simulink library "IOlib"  (R2014a)
settings: Solver=ode45  SolverMode=SingleTasking  StartTime=0.0  StopTime=10.0  RelTol=1e-3
values from neighbouring files (symbols this model uses):
  tm = (tm_l + tm_r)./2    [AACplottingcode.m]    (also in AACplottingcode_Mzcurves.m = 0.0212; IMECE06plottingcode.m; If_alpha_tp_observer_shoreline.m)
  Ts = 0.002    [DSC_Control_Analysis.m]    (also in DSC_Control_Analysis_Exp.m; DSC_Speed_Control_Analysis.m; EC_params_nissan.m; Ext_MPCPara.m = SSD.Ts)
undefined symbols (not defined in the file or in its folder): Amps_per_volt, bs, Eff, eff, fs, gr, Js, Kf, Ki, kM, Kp, L, ljt, lma, lmt, lsa, R, rjt, rma, rmt, rsa
undefined symbols (not defined in the file): DataDescription
libraries: simulink x3, xpcdiamondlib x2, HardwareIO x2, NullHardware x1, PrerecordData x1, VehicleSimulation x1
(part 1 of 2)
settings Model: ExtModeAutoUpdateStatusClock=off  Creator=cgadda  LastModifiedBy=cbeal

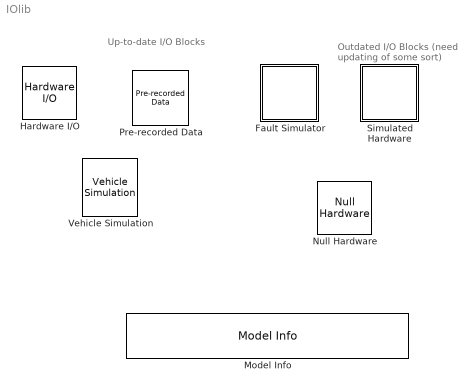
== system IOlib ==
  note: Up-to-date I/O Blocks
  note: Outdated I/O Blocks
      | (need updating of some sort)
  Fault Simulator : Subsystem
      mask init:
      | set_param('nissan_steer','StopTime','36000');
      | set_param('nissan_steer','StartTime','0');
      settings: OpenFcn=open_system([gcb '/Fault Simulator']);
      mask Display: disp('xPC');
  Hardware I/O : HardwareIO/Hardware I//O
  Model Info : simulink/Model-Wide Utilities/Model Info  InitialBlockCM=cvs  BlockCM=cvs  Frame=off  DisplayStringWithTags=|  HorizontalTextAlignment=Left  LeftAlignmentValue=0.02  SourceBlockDiagram=IOlib  TagMaxNumber=20
      | Last saved on: %<LastModificationDate>
      | Save number: %<ModelVersion>
      | Subversion: $Revision: 473 $
  Null Hardware : NullHardware/Null Hardware  SystemSampleTime=-1
  Pre-recorded Data : PrerecordData/Pre-recorded Data  filename=beal_2005-12-06_ab.mat  timeflag=off  starttime=0  stoptime=0
  Simulated Hardware : Subsystem  mask{stepsize=100, v=10, UseRealData=on, filename=/users/cgadda/nissan test data/Moffett1/gerdes_2004-12-11_a.mat}
      mask prompts: stepsize "Handwheel step steer magnitude (deg):"; v "Vehicle speed:"; UseRealData "Use pre-recorded driver input:"; filename "Pre-recorded data filename:"
      mask help:
      | This block provides a simulated hardware model.
      |
      | The driver command (speed and handwheel angle) is a step steer at constant speed.  The speed and magnitude of the manuever can be specified below.  Alternatively, the driver command can be taken from a pre-recorded data file.
      |
      | Note: when using this block, you MUST use a variable step size solver such as ode23.
      mask init:
      | p1_params
      | 
      | if(strcmp(filename,'-')|~UseRealData)
      | 	y=ones(1,18);
      | 	t=0;
      | 	DataDescription(1).name='Handwheel';
      | 	DataDescription(1).size=1;
      | 	DataDescription(2).name='GPS';
      | 	DataDescription(2).size=17;
      | else
      | 	load(filename);
      | end
      | 	
      | if(~(exist('DataDescription')&exist('y')&exist('t')))
      | 	error('Invalid data file.');
      | end
      mask Callback UseRealData:
      | if(strcmp(get_param(gcbh,'UseRealData'),'on')),
      | 	set_param(gcbh,'MaskEnables',{'off' 'off' 'on' 'on'});
      | else
      | 	set_param(gcbh,'MaskEnables',{'on' 'on' 'on' 'off'});
      | end
      mask Display: disp('Sim');
  Vehicle Simulation : VehicleSimulation/Vehicle Simulation  InitPosE=0  InitPosN=0  InitYawAngle=0  CruiseEnableTime=1  AutoSteerEnable=on  FaultEnable=off  HWHALEnable=off  TwoWheelEnable=on  DiffDriveEnable=off

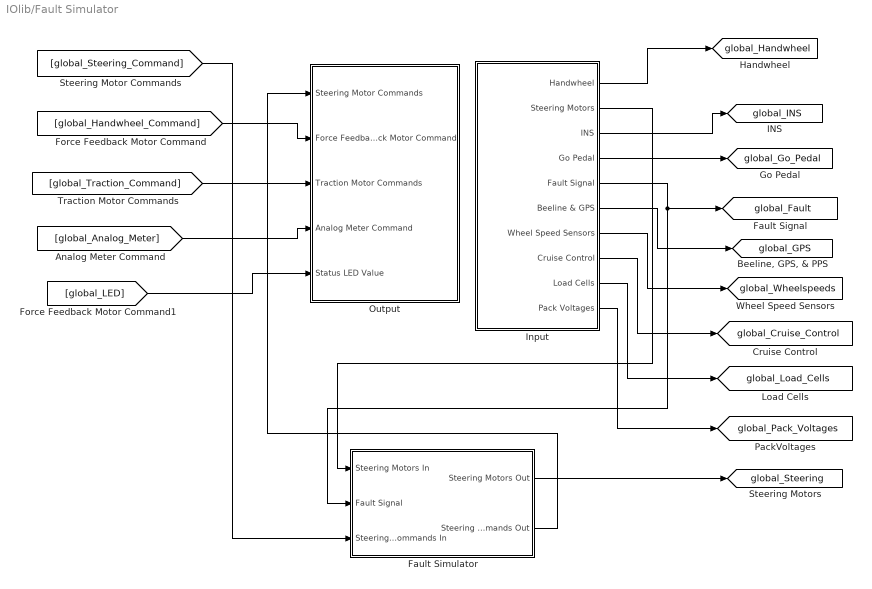
== system IOlib/Fault Simulator ==
  Fault Simulator : Subsystem  mask{fault=Current sensor, magnitude=0}
      mask prompts: fault "Type of fault"
      mask init:
      | switch(fault)
      | 	case 1
      | 		current=magnitude;
      | 		steer=0;
      | 	case 2
      | 		current=0;
      | 		steer=magnitude;
      | end
      mask TypeOptions fault: Current sensor | Steer angle sensor
  Input : Subsystem
  Output : Subsystem
  tag scope: global_Cruise_Control=global, global_Fault=global, global_GPS=global, global_Go_Pedal=global, global_Handwheel=global, global_INS=global, global_Load_Cells=global, global_Pack_Voltages=global, global_Steering=global, global_Wheelspeeds=global
  wires:
  Input/10(Pack Voltages) -> [global_Pack_Voltages]
  Input/9(Load Cells) -> [global_Load_Cells]
  [global_Traction_Command] -> Output/3(Traction Motor Commands)
  [global_Analog_Meter] -> Output/4(Analog Meter Command)
  [global_Steering_Command] -> Fault Simulator/3(Steering Motor Commands In)
  [global_Handwheel_Command] -> Output/2(Force Feedback Motor Command)
  [global_LED] -> Output/5(Status LED Value)
  Input/1(Handwheel) -> [global_Handwheel]
  Input/2(Steering Motors) -> Fault Simulator/1(Steering Motors In)
  Input/3(INS) -> [global_INS]
  Input/4(Go Pedal) -> [global_Go_Pedal]
  Input/5(Fault Signal) -> [global_Fault], Fault Simulator/2(Fault Signal)
  Input/6(Beeline & GPS) -> [global_GPS]
  Input/7(Wheel Speed Sensors) -> [global_Wheelspeeds]
  Input/8(Cruise Control) -> [global_Cruise_Control]
  Fault Simulator/1(Steering Motors Out) -> [global_Steering]
  Fault Simulator/2(Steering Motor Commands Out) -> Output/1(Steering Motor Commands)

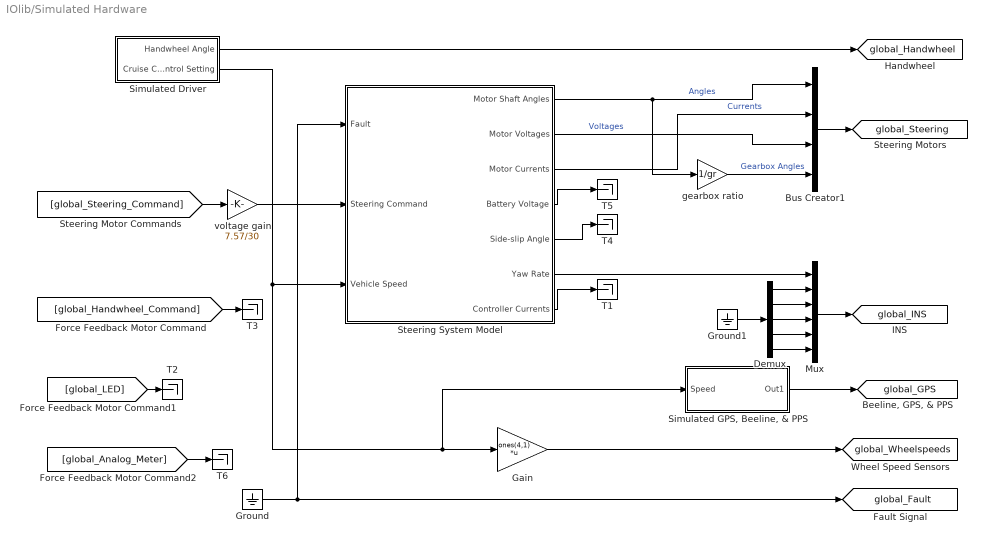
== system IOlib/Simulated Hardware ==
  Bus Creator1 : BusCreator
  Demux : Demux  Outputs=5
  Gain : Gain  Gain=ones(4,1)  Multiplication=Matrix(K*u)  SaturateOnIntegerOverflow=on  OutDataTypeStr=Inherit: Same as input  ParamDataTypeStr=Inherit: Same as input
  Ground : Ground
  Ground1 : Ground
  Mux : Mux  Inputs=6
  Simulated Driver : Subsystem
  "Simulated GPS, Beeline, & PPS" : Subsystem
  Steering System Model : Subsystem
  T{1..6} (6 alike) : Terminator
  gearbox ratio : Gain  Gain=1/gr  SaturateOnIntegerOverflow=on  OutDataTypeStr=Inherit: Same as input  ParamDataTypeStr=Inherit: Same as input
  voltage gain : Gain  Gain=7.57/30  SaturateOnIntegerOverflow=on  OutDataTypeStr=Inherit: Same as input  ParamDataTypeStr=Inherit: Same as input
  tag scope: global_Fault=global, global_GPS=global, global_Handwheel=global, global_INS=global, global_Steering=global, global_Wheelspeeds=global
  wires:
  voltage gain/1 -> Steering System Model/2(Steering Command)
  [global_Steering_Command] -> voltage gain/1
  [global_Analog_Meter] -> T6/1
  Steering System Model/4(Battery Voltage) -> T5/1
  Steering System Model/5(Side-slip Angle) -> T4/1
  [global_LED] -> T2/1
  Gain/1 -> [global_Wheelspeeds]
  [global_Handwheel_Command] -> T3/1
  Bus Creator1/1 -> [global_Steering]
  Steering System Model/1(Motor Shaft Angles) -> Bus Creator1/1, gearbox ratio/1  "Angles"
  Simulated Driver/1(Handwheel Angle) -> [global_Handwheel]
  gearbox ratio/1 -> Bus Creator1/4  "Gearbox Angles"
  Steering System Model/3(Motor Currents) -> Bus Creator1/2  "Currents"
  Steering System Model/2(Motor Voltages) -> Bus Creator1/3  "Voltages"
  Simulated Driver/2(Cruise Control Setting) -> "Simulated GPS, Beeline, & PPS"/1(Speed), Gain/1, Steering System Model/3(Vehicle Speed)
  Mux/1 -> [global_INS]
  Steering System Model/6(Yaw Rate) -> Mux/1
  Ground/1 -> [global_Fault], Steering System Model/1(Fault)
  Steering System Model/7(Controller Currents) -> T1/1
  "Simulated GPS, Beeline, & PPS"/1(Out1) -> [global_GPS]
  Demux/1 -> Mux/2
  Demux/5 -> Mux/6
  Demux/2 -> Mux/3
  Demux/3 -> Mux/4
  Demux/4 -> Mux/5
  Ground1/1 -> Demux/1

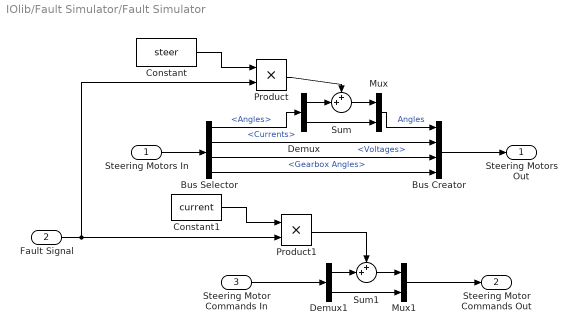
== system IOlib/Fault Simulator/Fault Simulator ==
  Steering Motors In : Inport
  Fault Signal : Inport  Port=2
  Steering Motor Commands In : Inport  Port=3
  Bus Creator : BusCreator
  Bus Selector : BusSelector  OutputSignals=Angles,Currents,Voltages,Gearbox Angles
  Constant : Constant  Value=steer
  Constant1 : Constant  Value=current
  Demux : Demux  Outputs=2
  Demux1 : Demux  Outputs=2
  Mux : Mux  Inputs=2
  Mux1 : Mux  Inputs=2
  Product : Product  RndMeth=Zero
  Product1 : Product  RndMeth=Zero
  Sum : Sum  Inputs=++|
  Sum1 : Sum  Inputs=++|
  Steering Motors Out : Outport
  Steering Motor Commands Out : Outport  Port=2
  wires:
  Bus Selector/4 -> Bus Creator/4  "<Gearbox Angles>"
  Bus Selector/3 -> Bus Creator/3  "<Voltages>"
  Bus Selector/2 -> Bus Creator/2  "<Currents>"
  Steering Motors In/1 -> Bus Selector/1
  Bus Creator/1 -> Steering Motors Out/1
  Demux/1 -> Sum/2
  Sum/1 -> Mux/1
  Demux/2 -> Mux/2
  Bus Selector/1 -> Demux/1  "<Angles>"
  Mux/1 -> Bus Creator/1  "Angles"
  Constant/1 -> Product/1
  Product/1 -> Sum/1
  Steering Motor Commands In/1 -> Demux1/1
  Demux1/1 -> Sum1/2
  Sum1/1 -> Mux1/1
  Demux1/2 -> Mux1/2
  Mux1/1 -> Steering Motor Commands Out/1
  Constant1/1 -> Product1/1
  Product1/1 -> Sum1/1
  Fault Signal/1 -> Product1/2, Product/2

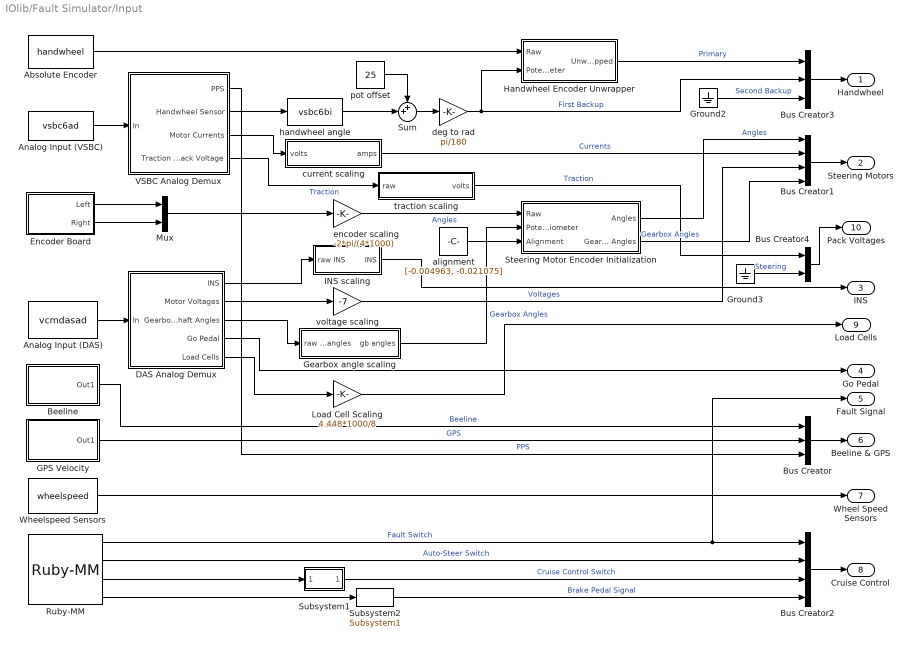
== system IOlib/Fault Simulator/Input ==
  Absolute Encoder : S-Function  FunctionName=handwheel  Parameters=Ts  EnableBusSupport=off
  Analog Input (DAS) : S-Function  FunctionName=vcmdasad  Parameters=numChannels, inputVec, sampleTime  EnableBusSupport=off  mask{numChannels=16, inputVec=[4 4 4 4 4 4 4 4 4 4 4 4 4 4 4 4], sampleTime=Ts}
      mask prompts: sampleTime "sample_time"
  Analog Input (VSBC) : S-Function  FunctionName=vsbc6ad  Parameters=numChannels,inpRange,sampTime  EnableBusSupport=off  mask{numChannels=8, inpRange=[4 4 1 1 1 3 3 2], sampTime=Ts}
      mask prompts: numChannels "Number of Channels"; inpRange "Analog Input Range (1: +5; 2: +10; 3: +-5; 4: +-10)"; sampTime "Sampling Time"
  Beeline : Subsystem
      mask Display: disp('beeline');
  Bus Creator : BusCreator  Inputs=3
  Bus Creator1 : BusCreator
  Bus Creator2 : BusCreator
  Bus Creator3 : BusCreator  Inputs=3
  Bus Creator4 : BusCreator  Inputs=2
  DAS Analog Demux : Subsystem
  Encoder Board : Subsystem
  GPS Velocity : Subsystem
      mask Display: disp('OEM4');
  Gearbox angle scaling : Subsystem
  Ground2 : Ground
  Ground3 : Ground
  Handwheel Encoder Unwrapper : Subsystem
  INS scaling : Subsystem
  Load Cell Scaling : Gain  Gain=4.448*1000/8  SaturateOnIntegerOverflow=on  OutDataTypeStr=Inherit: Same as input  ParamDataTypeStr=Inherit: Same as input
  Mux : Mux  Inputs=2
  Ruby-MM : xpcdiamondlib/Digital Input/Ruby-MM   channel=[5 6 7 8]  port=A  chip=1  sampletime=Ts  baseaddress=0x300
  Steering Motor Encoder Initialization : Subsystem
      mask init:
      | p1_params
  Subsystem1 : Subsystem
      mask Display: disp('!');
  Subsystem2 : HardwareIO/Hardware I//O/Input/Subsystem1  SystemSampleTime=-1
  Sum : Sum  Inputs=++|
  VSBC Analog Demux : Subsystem
  Wheelspeed Sensors : S-Function  FunctionName=wheelspeed  Parameters=Ts  EnableBusSupport=off
  alignment : Constant  Value=[-0.004963, -0.021075]
  current scaling : Subsystem
  deg to rad : Gain  Gain=pi/180  SaturateOnIntegerOverflow=on  OutDataTypeStr=Inherit: Same as input  ParamDataTypeStr=Inherit: Same as input
  encoder scaling : Gain  Gain=-2*pi/(4*1000)  SaturateOnIntegerOverflow=on  OutDataTypeStr=Inherit: Same as input  ParamDataTypeStr=Inherit: Same as input
  handwheel angle : S-Function  FunctionName=vsbc6bi  Parameters=sampTime  EnableBusSupport=off  mask{sampTime=Ts}
      mask prompts: sampTime "Sampling Time"
  pot offset : Constant  Value=25
  traction scaling : Subsystem
  voltage scaling : Gain  Gain=-7  SaturateOnIntegerOverflow=on  OutDataTypeStr=Inherit: Same as input  ParamDataTypeStr=Inherit: Same as input
  Handwheel : Outport
  Steering Motors : Outport  Port=2
  INS : Outport  Port=3
  Go Pedal : Outport  Port=4
  Fault Signal : Outport  Port=5
  Beeline & GPS : Outport  Port=6
  Wheel Speed Sensors : Outport  Port=7
  Cruise Control : Outport  Port=8
  Load Cells : Outport  Port=9
  Pack Voltages : Outport  Port=10
  wires:
  Handwheel Encoder Unwrapper/1(Unwrapped) -> Bus Creator3/1  "Primary"
  VSBC Analog Demux/4(Traction Pack Voltage) -> traction scaling/1(raw)  "Traction"
  Ground3/1 -> Bus Creator4/2  "Steering"
  Bus Creator4/1 -> Pack Voltages/1
  Load Cell Scaling/1 -> Load Cells/1
  DAS Analog Demux/5(Load Cells) -> Load Cell Scaling/1
  deg to rad/1 -> Handwheel Encoder Unwrapper/2(Potentiometer), Bus Creator3/2  "First Backup"
  Bus Creator3/1 -> Handwheel/1
  DAS Analog Demux/4(Go Pedal) -> Go Pedal/1
  Bus Creator2/1 -> Cruise Control/1
  DAS Analog Demux/2(Motor Voltages) -> voltage scaling/1
  voltage scaling/1 -> Bus Creator1/3  "Voltages"
  Mux/1 -> encoder scaling/1
  Encoder Board/2(Right) -> Mux/2
  Encoder Board/1(Left) -> Mux/1
  Analog Input (VSBC)/1 -> VSBC Analog Demux/1(In)
  VSBC Analog Demux/1(PPS) -> Bus Creator/3  "PPS"
  VSBC Analog Demux/2(Handwheel Sensor) -> handwheel angle/1
  Beeline/1(Out1) -> Bus Creator/1  "Beeline"
  GPS Velocity/1(Out1) -> Bus Creator/2  "GPS"
  Bus Creator/1 -> Beeline & GPS/1
  Bus Creator1/1 -> Steering Motors/1
  Wheelspeed Sensors/1 -> Wheel Speed Sensors/1
  VSBC Analog Demux/3(Motor Currents) -> current scaling/1(volts)
  current scaling/1(amps) -> Bus Creator1/2  "Currents"
  INS scaling/1(INS) -> INS/1
  DAS Analog Demux/1(INS) -> INS scaling/1(raw INS)
  Analog Input (DAS)/1 -> DAS Analog Demux/1(In)
  DAS Analog Demux/3(Gearbox Shaft Angles) -> Gearbox angle scaling/1(raw gb angles)
  Gearbox angle scaling/1(gb angles) -> Steering Motor Encoder Initialization/2(Potentiometer)  "Gearbox Angles"
  Subsystem1/1(Out1) -> Bus Creator2/3  "Cruise Control Switch"
  Subsystem2/1 -> Bus Creator2/4  "Brake Pedal Signal"
  encoder scaling/1 -> Steering Motor Encoder Initialization/1(Raw)  "Angles"
  Absolute Encoder/1 -> Handwheel Encoder Unwrapper/1(Raw)
  Ground2/1 -> Bus Creator3/3  "Second Backup"
  handwheel angle/1 -> Sum/2
  pot offset/1 -> Sum/1
  Sum/1 -> deg to rad/1
  Steering Motor Encoder Initialization/1(Angles) -> Bus Creator1/1  "Angles"
  alignment/1 -> Steering Motor Encoder Initialization/3(Alignment)
  Steering Motor Encoder Initialization/2(Gearbox Angles) -> Bus Creator1/4  "Gearbox Angles"
  Ruby-MM/3 -> Subsystem1/1(In1)
  Ruby-MM/4 -> Subsystem2/1
  Ruby-MM/2 -> Bus Creator2/2  "Auto-Steer Switch"
  Ruby-MM/1 -> Bus Creator2/1, Fault Signal/1  "Fault Switch"
  traction scaling/1(volts) -> Bus Creator4/1  "Traction"

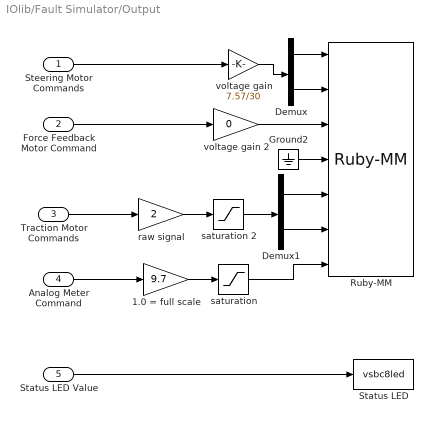
== system IOlib/Fault Simulator/Output ==
  Steering Motor Commands : Inport
  Force Feedback Motor Command : Inport  Port=2
  Traction Motor Commands : Inport  Port=3
  Analog Meter Command : Inport  Port=4
  Status LED Value : Inport  Port=5
  1.0 = full scale : Gain  Gain=9.7  SaturateOnIntegerOverflow=on  OutDataTypeStr=Inherit: Same as input  ParamDataTypeStr=Inherit: Same as input
  Demux : Demux  Outputs=2
  Demux1 : Demux  Outputs=2
  Ground2 : Ground
  "Ruby-MM " : xpcdiamondlib/D//A/Ruby-MM   channel=[1 2 3 4 5 6 7]  range0=+-10  range1=+-10  reset=[1 1 1 1 1 1 1]  initValue=[0 0 0 0 0 0 0]  st=Ts  baseaddress=0x300
  Status LED : S-Function  FunctionName=vsbc8led  EnableBusSupport=off
  raw signal : Gain  Gain=2  SaturateOnIntegerOverflow=on  OutDataTypeStr=Inherit: Same as input  ParamDataTypeStr=Inherit: Same as input
  saturation : Saturate  UpperLimit=11  LowerLimit=0
  saturation 2 : Saturate  UpperLimit=5.5  LowerLimit=2
  voltage gain : Gain  Gain=7.57/30  SaturateOnIntegerOverflow=on  OutDataTypeStr=Inherit: Same as input  ParamDataTypeStr=Inherit: Same as input
  voltage gain 2 : Gain  Gain=0  SaturateOnIntegerOverflow=on  OutDataTypeStr=Inherit: Same as input  ParamDataTypeStr=Inherit: Same as input
  wires:
  voltage gain 2/1 -> "Ruby-MM "/3
  Force Feedback Motor Command/1 -> voltage gain 2/1
  raw signal/1 -> saturation 2/1
  saturation 2/1 -> Demux1/1
  saturation/1 -> "Ruby-MM "/7
  Demux1/2 -> "Ruby-MM "/6
  Steering Motor Commands/1 -> voltage gain/1
  voltage gain/1 -> Demux/1
  1.0 = full scale/1 -> saturation/1
  Ground2/1 -> "Ruby-MM "/4
  Demux/2 -> "Ruby-MM "/2
  Demux/1 -> "Ruby-MM "/1
  Status LED Value/1 -> Status LED/1
  Demux1/1 -> "Ruby-MM "/5
  Traction Motor Commands/1 -> raw signal/1
  Analog Meter Command/1 -> 1.0 = full scale/1

== system IOlib/Simulated Hardware/Simulated Driver ==
  Automatic Manual Switch : Subsystem  AncestorBlock=simulink/Signal Routing/Manual Switch  mask(Manual Switch){sw=~UseRealData, action=0}
      mask prompts: sw "Current setting:"
      mask help: Output toggles between two inputs by double-clicking on the block.
      mask init:
      | %manswitch;
      | 
      | blk=gcbh;
      | BlockPos=get_param(blk,'Position');
      | Width=BlockPos(3)-BlockPos(1);
      | Height=BlockPos(4)-BlockPos(2);
      | %updown=~xor(action,sw);
      | updown=~sw;
      | 
      | PortInfo=get_param(blk,'PortConnectivity');
      | PortPos=cat(1,PortInfo.Position);
      | % Port locations in global Simulink coordinates
      | x=PortPos(:,1);
      | y=PortPos(:,2);
      | % Move locations inside of block icon (still global coordinates)
      | x = x + 5*(x < BlockPos(1)) - 5*(x > BlockPos(3));
      | y = y + 5*(y < BlockPos(2)) - 5*(y > BlockPos(4));
      | % Convert to plot coordinates
      | x = x - BlockPos(1);
      | y = BlockPos(4) - y;
      | PortPos=[x y];
      | 
      | Radius=ceil(min(Height,Width)/25);
      | LineLength=min(6,10*Radius/3);
      | Offset=Radius+LineLength;
      | 
      | centers=PortPos+Offset*[[ones(1,4) -1 -1]' zeros(6,1)];
      | 
      | t=(0:20)/20*2*pi;
      | CircX=cos(t)*Radius;
      | CircY=sin(t)*Radius;
      | 
      | AllCircX=[CircX+centers(1,1) NaN ...
      | 		  CircX+centers(2,1) NaN ...
      | 		  CircX+centers(3,1) NaN ...
      | 		  CircX+centers(4,1) NaN ...
      | 		  CircX+centers(5,1) NaN ...
      | 		  CircX+centers(6,1)];
      | AllCircY=[CircY+centers(1,2) NaN ...
      | 		  CircY+centers(2,2) NaN ...
      | 		  CircY+centers(3,2) NaN ...
      | 		  CircY+centers(4,2) NaN ...
      | 		  CircY+centers(5,2) NaN ...
      | 		  CircY+centers(6,2)];
      | 
      | LLX=[PortPos(1,1) centers(1,1)-Radius NaN ...
      |      PortPos(2,1) centers(2,1)-Radius NaN ...
      | 	 PortPos(3,1) centers(3,1)-Radius NaN ...
      | 	 PortPos(4,1) centers(4,1)-Radius NaN ...
      | 	 PortPos(5,1) centers(5,1)+Radius NaN ...
      | 	 PortPos(6,1) centers(6,1)+Radius];
      | LLY=[PortPos(1,2) centers(1,2) NaN ...
      | 	 PortPos(2,2) centers(2,2) NaN ...
      | 	 PortPos(3,2) centers(3,2) NaN ...
      | 	 PortPos(4,2) centers(4,2) NaN ...
      | 	 PortPos(5,2) centers(5,2) NaN ...
      | 	 PortPos(6,2) centers(6,2)];
      | 
      | if(updown~=0 & updown~=1)
      | 	error(sprintf('Something isn''t right. %d %d',updown,action));
      | end
      | 
      | FlapsX=[centers(5,1) centers(1+updown,1) NaN ...
      | 	    centers(6,1) centers(3+updown,1)];
      | FlapsY=[centers(5,2) centers(1+updown,2) NaN ...
      | 	    centers(6,2) centers(3+updown,2)];
      | 	
      | m=[AllCircX NaN LLX NaN FlapsX];
      | n=[AllCircY NaN LLY NaN FlapsY];
      mask Help: This block implements a manual switch.
      mask Display: plot(m,n);
  From Workspace : FromWorkspace  VariableName=[t y]  SampleTime=0  OutputAfterFinalValue=Setting to zero
  Named Demux : S-Function  FunctionName=nameddemux  Parameters=outputcount, outputsizes, outputindices, inputsize  EnableBusSupport=off  mask{desc=DataDescription, signals={'Handwheel' 'GPS'}}
      mask prompts: desc "Data description function name"; signals "Signal names"
      mask help:
      | Combines input signals into a single output vector, according to a structure that provides the names and sizes of each signal.
      |
      | The parameter below should be set to the name of a function which returns a 1xN structure array, where N is the number of input signals.  The structure should contain fields "size" which specifies the width of the input signal, and "name" which specifies its name.
      mask init:
      | outputcount=length(signals);
      | inputsize=sum([desc.size]);
      | 
      | indices=[1 cumsum([desc.size])+1];
      | 
      | if((outputcount<1)|(outputcount>50))
      | 	error('Inappropriate number of outputs.');
      | end
      | 
      | y=ones(1,outputcount);
      | 
      | for indx=1:outputcount,
      |     sig=signals{indx};
      | 	sigi=find(strcmp(sig,{desc.name}));
      |     if (length(sigi)==0)
      |         error(['Unable to find signal named "' sig '".']);
      |     end
      |     y(indx)=sigi;
      | end
      | 		
      | outputsizes=[desc(y).size];
      | outputindices=indices(y);
      | 
      | x=min(outputcount*ones(1,50),1:50);
      mask Display:
      | port_label('output',x(1),desc(y(x(1))).name);
      | port_label('output',x(2),desc(y(x(2))).name);
  Select: Speed : Subsystem  mask{indices=13, width=17}
      mask prompts: indices "Signal indices"; width "Input width"
      mask init:
      | ic=length(indices);
      | 
      | K=zeros(ic,width);
      | 
      | for ii=1:ic,
      | 	K(ii,indices(ii))=1;
      | end
      mask Display: disp(indices)
  Step : Step  Time=.5  After=stepsize*(pi/180)  SampleTime=0
  Vehicle Speed : Constant  Value=v
  Handwheel Angle : Outport
  Cruise Control Setting : Outport  Port=2
  wires:
  Select: Speed/1(Out1) -> Automatic Manual Switch/4(4)
  Named Demux/2 -> Select: Speed/1(In1)
  From Workspace/1 -> Named Demux/1
  Automatic Manual Switch/1(Out1) -> Handwheel Angle/1
  Named Demux/1 -> Automatic Manual Switch/2(2)
  Step/1 -> Automatic Manual Switch/1(1)
  Automatic Manual Switch/2(Out2) -> Cruise Control Setting/1
  Vehicle Speed/1 -> Automatic Manual Switch/3(3)

== system IOlib/Simulated Hardware/Simulated GPS, Beeline, & PPS ==
  Speed : Inport
  Bus Creator : BusCreator  Inputs=3
  Constant2 : Constant  Value=zeros(16,1)
  Demux : Demux  Outputs=16
  Mux : Mux  Inputs=10
  Mux1 : Mux  Inputs=6
  Pulse Generator : DiscretePulseGenerator  PulseType=Time based  Amplitude=5  Period=1  PulseWidth=50
  Terminator2 : Terminator
  Out1 : Outport
  wires:
  Speed/1 -> Mux1/3  "Horizontal Speed"
  Bus Creator/1 -> Out1/1
  Mux1/1 -> Bus Creator/2  "GPS"
  Mux/1 -> Bus Creator/1  "Beeline"
  Pulse Generator/1 -> Bus Creator/3  "PPS"
  Demux/10 -> Mux/10  "Velocity Status"
  Demux/9 -> Mux/9  "Vertical Speed"
  Demux/8 -> Mux/8  "Direction"
  Demux/7 -> Mux/7  "Horizontal Speed"
  Demux/6 -> Mux/6  "Latency"
  Demux/5 -> Mux/5  "UTC 2"
  Demux/4 -> Mux/4  "Attitude Status"
  Demux/3 -> Mux/3  "Roll Angle"
  Demux/2 -> Mux/2  "Yaw Angle"
  Demux/1 -> Mux/1  "UTC 1"
  Demux/16 -> Mux1/6  "Status"
  Demux/15 -> Mux1/5  "Vertical Speed"
  Demux/14 -> Mux1/4  "Direction"
  Demux/12 -> Mux1/2  "Latency"
  Demux/11 -> Mux1/1  "UTC"
  Constant2/1 -> Demux/1  "Beeline"
  Demux/13 -> Terminator2/1

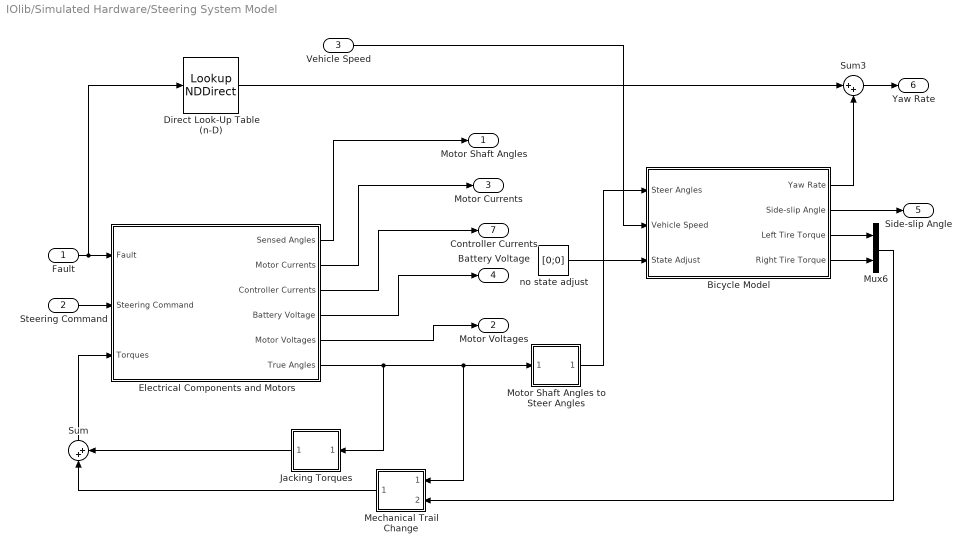
== system IOlib/Simulated Hardware/Steering System Model ==
  Fault : Inport
  Steering Command : Inport  Port=2
  Vehicle Speed : Inport  Port=3
  Bicycle Model : Subsystem
  Direct Look-Up Table (n-D) : LookupNDDirect  NumberOfTableDimensions=1  Table=[0 0 0 0 0 .01]
  Electrical Components and Motors : Subsystem
  Jacking Torques : Subsystem
      mask init:
      | % Generate the lookup tables
      | p1_params
      | nissan_steer_lookup_data
      mask Display: disp('.')
  Mechanical Trail Change : Subsystem
      mask init:
      | % Generate the lookup tables
      | p1_params
      | nissan_steer_lookup_data
      mask Display: disp('.')
  Motor Shaft Angles to Steer Angles : Subsystem
      mask init:
      | % Generate the lookup tables
      | p1_params
      | nissan_steer_lookup_data
      mask Display: disp('.')
  Mux6 : Mux  Inputs=2
  Sum : Sum  Inputs=|++  SaturateOnIntegerOverflow=on
  Sum3 : Sum  Inputs=|++  SaturateOnIntegerOverflow=on
  no state adjust : Constant  Value=[0;0]
  Motor Shaft Angles : Outport
  Motor Voltages : Outport  Port=2
  Motor Currents : Outport  Port=3
  Battery Voltage : Outport  Port=4
  Side-slip Angle : Outport  Port=5
  Yaw Rate : Outport  Port=6
  Controller Currents : Outport  Port=7
  wires:
  Sum/1 -> Electrical Components and Motors/3(Torques)
  Steering Command/1 -> Electrical Components and Motors/2(Steering Command)
  Mechanical Trail Change/1(Actual Aligning Torques) -> Sum/1
  Mux6/1 -> Mechanical Trail Change/2(Nominal Aligning Torques)
  Jacking Torques/1(Jacking Torques) -> Sum/2
  Motor Shaft Angles to Steer Angles/1(Steer Angles) -> Bicycle Model/1(Steer Angles)
  Electrical Components and Motors/6(True Angles) -> Jacking Torques/1(Motor Shaft Angles), Motor Shaft Angles to Steer Angles/1(Motor Shaft Angles), Mechanical Trail Change/1(Motor Shaft Angles)
  Electrical Components and Motors/1(Sensed Angles) -> Motor Shaft Angles/1
  no state adjust/1 -> Bicycle Model/3(State Adjust)
  Electrical Components and Motors/5(Motor Voltages) -> Motor Voltages/1
  Electrical Components and Motors/4(Battery Voltage) -> Battery Voltage/1
  Electrical Components and Motors/3(Controller Currents) -> Controller Currents/1
  Direct Look-Up Table (n-D)/1 -> Sum3/1
  Fault/1 -> Electrical Components and Motors/1(Fault), Direct Look-Up Table (n-D)/1
  Electrical Components and Motors/2(Motor Currents) -> Motor Currents/1
  Sum3/1 -> Yaw Rate/1
  Vehicle Speed/1 -> Bicycle Model/2(Vehicle Speed)
  Bicycle Model/4(Right Tire Torque) -> Mux6/2
  Bicycle Model/3(Left Tire Torque) -> Mux6/1
  Bicycle Model/2(Side-slip Angle) -> Side-slip Angle/1
  Bicycle Model/1(Yaw Rate) -> Sum3/2

== system IOlib/Fault Simulator/Input/Beeline ==
  Beeline : S-Function  FunctionName=beeline  Parameters=Ts  EnableBusSupport=off
  Demux : Demux  Outputs=10
  Mux : Mux  Inputs=10
  Out1 : Outport
  wires:
  Demux/10 -> Mux/10  "Velocity Status"
  Demux/9 -> Mux/9  "Vertical Speed"
  Demux/8 -> Mux/8  "Direction"
  Demux/7 -> Mux/7  "Horizontal Speed"
  Demux/6 -> Mux/6  "Latency"
  Demux/5 -> Mux/5  "UTC 2"
  Demux/4 -> Mux/4  "Attitude Status"
  Demux/3 -> Mux/3  "Roll Angle"
  Demux/2 -> Mux/2  "Yaw Angle"
  Demux/1 -> Mux/1  "UTC 1"
  Mux/1 -> Out1/1
  Beeline/1 -> Demux/1

== system IOlib/Fault Simulator/Input/DAS Analog Demux ==
  In : Inport
  Demux : Demux  Outputs=16
  Mux : Mux  Inputs=9
  Mux1 : Mux  Inputs=2
  Mux2 : Mux  Inputs=2
  Mux3 : Mux  Inputs=2
  INS : Outport
  Motor Voltages : Outport  Port=2
  Gearbox Shaft Angles : Outport  Port=3
  Go Pedal : Outport  Port=4
  Load Cells : Outport  Port=5
  wires:
  Demux/10 -> Go Pedal/1
  Mux3/1 -> Load Cells/1
  Demux/16 -> Mux2/2
  Demux/15 -> Mux2/1
  Demux/2 -> Mux/2
  Demux/14 -> Mux1/2
  Demux/13 -> Mux1/1
  Mux1/1 -> Motor Voltages/1
  Mux/1 -> INS/1
  Demux/9 -> Mux/9
  Demux/8 -> Mux/8
  Demux/7 -> Mux/7
  Demux/6 -> Mux/6
  Demux/5 -> Mux/5
  Demux/4 -> Mux/4
  Demux/3 -> Mux/3
  Demux/1 -> Mux/1
  In/1 -> Demux/1
  Mux2/1 -> Gearbox Shaft Angles/1
  Demux/11 -> Mux3/2
  Demux/12 -> Mux3/1

== system IOlib/Fault Simulator/Input/Encoder Board ==
  "encoder board " : S-Function  FunctionName=UltimateEncoder  Parameters=TSamp,NC,BA,[R1 R2 R3 R4 R5 R6 ]  EnableBusSupport=off  mask{TSamp=Ts, BA=528, NC=2, R1=on, R2=on, R3=off, R4=off, R5=off, R6=off}
      mask prompts: TSamp "Sampling Rate"; BA "Base Adress (Base 10)"; NC "Number of Channels"; R1 "Unwrap Channel 1"; R2 "Unwrap Channel 2"; R3 "Unwrap Channel 3"; R4 "Unwrap Channel 4"; R5 "Unwrap Channel 5"; R6 "Unwrap Channel 6"
  reset : Constant  Value=[1 1]
  Left : Outport
  Right : Outport  Port=2
  wires:
  reset/1 -> "encoder board "/1
  "encoder board "/1 -> Left/1
  "encoder board "/2 -> Right/1

== system IOlib/Fault Simulator/Input/GPS Velocity ==
  Demux : Demux  Outputs=6
  GPS Velocity : S-Function  FunctionName=rs232_OEM4_vel  Parameters=Ts  EnableBusSupport=off
  Mux : Mux  Inputs=6
  Out1 : Outport
  wires:
  GPS Velocity/1 -> Demux/1
  Mux/1 -> Out1/1
  Demux/1 -> Mux/1  "UTC"
  Demux/2 -> Mux/2  "Latency"
  Demux/3 -> Mux/3  "Horizontal Speed"
  Demux/4 -> Mux/4  "Direction"
  Demux/5 -> Mux/5  "Vertical Speed"
  Demux/6 -> Mux/6  "Status"

== system IOlib/Fault Simulator/Input/Gearbox angle scaling ==
  raw gb angles : Inport
  Alignment : Constant  Value=[ 2.461417; 2.039667 ]  VectorParams1D=off
  Gain : Gain  Gain=[ -0.805*1.063; -0.795*0.926]  SaturateOnIntegerOverflow=on  OutDataTypeStr=Inherit: Same as input  ParamDataTypeStr=Inherit: Same as input
  Radians Alignment : Constant  Value=[ -.440337; 1.010775]  VectorParams1D=off
  Sum : Sum  Inputs=|+-  SaturateOnIntegerOverflow=on
  Sum1 : Sum  Inputs=++|  SaturateOnIntegerOverflow=on
  gb angles : Outport
  wires:
  Sum1/1 -> gb angles/1
  Gain/1 -> Sum1/2
  Radians Alignment/1 -> Sum1/1
  raw gb angles/1 -> Sum/1
  Alignment/1 -> Sum/2
  Sum/1 -> Gain/1

== system IOlib/Fault Simulator/Input/Handwheel Encoder Unwrapper ==
  Raw : Inport
  Potentiometer : Inport  Port=2
  Compare To Constant : simulink/Logic and Bit Operations/Compare To Constant  relop=<=  const=-3  OutDataTypeStr=boolean  ZeroCross=off
  Compare To Constant1 : simulink/Logic and Bit Operations/Compare To Constant  relop=>=  const=3  OutDataTypeStr=boolean  ZeroCross=off
  Gain : Gain  Gain=2*pi
  Gain1 : Gain  Gain=-2*pi
  Sum : Sum  Inputs=|++  SaturateOnIntegerOverflow=on
  Sum1 : Sum  Inputs=-+|  SaturateOnIntegerOverflow=on
  Sum2 : Sum  Inputs=++|  SaturateOnIntegerOverflow=on
  bool to double : DataTypeConversion  OutDataTypeStr=double
  "bool to double, too" : DataTypeConversion  OutDataTypeStr=double
  Unwrapped : Outport
  wires:
  Sum/1 -> Unwrapped/1
  Raw/1 -> Sum/1, Sum1/1
  Potentiometer/1 -> Sum1/2
  Sum1/1 -> Compare To Constant1/1, Compare To Constant/1
  Compare To Constant1/1 -> bool to double/1
  Compare To Constant/1 -> "bool to double, too"/1
  Sum2/1 -> Sum/2
  bool to double/1 -> Gain/1
  Gain/1 -> Sum2/1
  "bool to double, too"/1 -> Gain1/1
  Gain1/1 -> Sum2/2

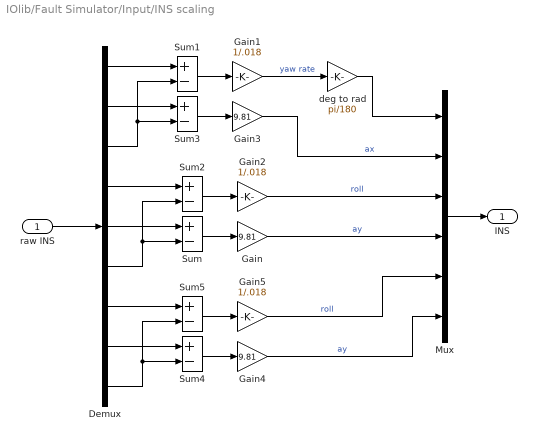
== system IOlib/Fault Simulator/Input/INS scaling ==
  raw INS : Inport
  Demux : Demux  Outputs=9
  Gain : Gain  Gain=9.81  SaturateOnIntegerOverflow=on  OutDataTypeStr=Inherit: Same as input  ParamDataTypeStr=Inherit: Same as input
  Gain1 : Gain  Gain=1/.018  SaturateOnIntegerOverflow=on  OutDataTypeStr=Inherit: Same as input  ParamDataTypeStr=Inherit: Same as input
  Gain2 : Gain  Gain=1/.018  SaturateOnIntegerOverflow=on  OutDataTypeStr=Inherit: Same as input  ParamDataTypeStr=Inherit: Same as input
  Gain3 : Gain  Gain=9.81  SaturateOnIntegerOverflow=on  OutDataTypeStr=Inherit: Same as input  ParamDataTypeStr=Inherit: Same as input
  Gain4 : Gain  Gain=9.81  SaturateOnIntegerOverflow=on  OutDataTypeStr=Inherit: Same as input  ParamDataTypeStr=Inherit: Same as input
  Gain5 : Gain  Gain=1/.018  SaturateOnIntegerOverflow=on  OutDataTypeStr=Inherit: Same as input  ParamDataTypeStr=Inherit: Same as input
  Mux : Mux  Inputs=6
  Sum{,1..5} (6 alike) : Sum  Inputs=+-  SaturateOnIntegerOverflow=on  InputSameDT=on  OutDataTypeStr=Inherit: Same as first input
  deg to rad : Gain  Gain=pi/180  SaturateOnIntegerOverflow=on  OutDataTypeStr=Inherit: Same as input  ParamDataTypeStr=Inherit: Same as input
  INS : Outport
  wires:
  Mux/1 -> INS/1
  deg to rad/1 -> Mux/1
  Demux/9 -> Sum4/2, Sum5/2
  Demux/5 -> Sum/1
  Demux/8 -> Sum4/1
  Demux/7 -> Sum5/1
  Sum4/1 -> Gain4/1
  Sum5/1 -> Gain5/1
  Gain4/1 -> Mux/6  "ay"
  Gain5/1 -> Mux/5  "roll"
  raw INS/1 -> Demux/1
  Sum/1 -> Gain/1
  Sum1/1 -> Gain1/1
  Sum2/1 -> Gain2/1
  Sum3/1 -> Gain3/1
  Gain/1 -> Mux/4  "ay"
  Gain1/1 -> deg to rad/1  "yaw rate"
  Gain2/1 -> Mux/3  "roll"
  Gain3/1 -> Mux/2  "ax"
  Demux/1 -> Sum1/1
  Demux/3 -> Sum1/2, Sum3/2
  Demux/2 -> Sum3/1
  Demux/4 -> Sum2/1
  Demux/6 -> Sum/2, Sum2/2

== system IOlib/Fault Simulator/Input/Steering Motor Encoder Initialization ==
  Raw : Inport
  Potentiometer : Inport  Port=2
  Alignment : Inport  Port=3
  Demux : Demux  Outputs=2
  Demux1 : Demux  Outputs=2
  Left : Subsystem
  Mux : Mux  Inputs=2
  Right : Subsystem
  Sum1 : Sum  Inputs=++|
  Sum2 : Sum  Inputs=|++
  gearbox ratio : Gain  Gain=gr  SaturateOnIntegerOverflow=on  OutDataTypeStr=Inherit: Same as input  ParamDataTypeStr=Inherit: Same as input
  gearbox ratio1 : Gain  Gain=gr  SaturateOnIntegerOverflow=on  OutDataTypeStr=Inherit: Same as input  ParamDataTypeStr=Inherit: Same as input
  Angles : Outport
  Gearbox Angles : Outport  Port=2
  wires:
  Demux1/2 -> Right/2(Potentiometer)
  Demux1/1 -> Left/2(Potentiometer)
  Demux/2 -> Right/1(Encoder)
  Demux/1 -> Left/1(Encoder)
  Left/1(Calibrated) -> Mux/1
  Potentiometer/1 -> gearbox ratio/1, Sum1/2
  Raw/1 -> Demux/1
  gearbox ratio/1 -> Demux1/1
  Right/1(Calibrated) -> Mux/2
  Mux/1 -> Sum2/1
  Sum2/1 -> Angles/1
  Alignment/1 -> gearbox ratio1/1, Sum1/1
  gearbox ratio1/1 -> Sum2/2
  Sum1/1 -> Gearbox Angles/1

== system IOlib/Fault Simulator/Input/Subsystem1 ==
  In1 : Inport
  Constant : Constant
  Sum : Sum  Inputs=+-|
  Out1 : Outport
  wires:
  Constant/1 -> Sum/1
  In1/1 -> Sum/2
  Sum/1 -> Out1/1

== system IOlib/Fault Simulator/Input/VSBC Analog Demux ==
  In : Inport
  Demux : Demux  Outputs=8
  Mux : Mux  Inputs=3
  Mux1 : Mux  Inputs=2
  T2 : Terminator
  PPS : Outport
  Handwheel Sensor : Outport  Port=2
  Motor Currents : Outport  Port=3
  Traction Pack Voltage : Outport  Port=4
  wires:
  Demux/8 -> Traction Pack Voltage/1
  Demux/1 -> PPS/1
  Demux/2 -> T2/1
  Demux/5 -> Mux/3
  Demux/4 -> Mux/2
  Demux/3 -> Mux/1
  Demux/6 -> Mux1/1
  Demux/7 -> Mux1/2
  In/1 -> Demux/1
  Mux/1 -> Handwheel Sensor/1
  Mux1/1 -> Motor Currents/1

== system IOlib/Fault Simulator/Input/current scaling ==
  volts : Inport
  Constant : Constant  Value=-5.39
  Sum : Sum  Inputs=|++  SaturateOnIntegerOverflow=on
  current scaling : Gain  Gain=30/7.5*3.3  SaturateOnIntegerOverflow=on  OutDataTypeStr=Inherit: Same as input  ParamDataTypeStr=Inherit: Same as input
  amps : Outport
  wires:
  Constant/1 -> Sum/2
  Sum/1 -> amps/1
  current scaling/1 -> Sum/1
  volts/1 -> current scaling/1

== system IOlib/Fault Simulator/Input/traction scaling ==
  raw : Inport
  Constant : Constant  Value=8.9342
  Constant1 : Constant  Value=127
  Sum : Sum  Inputs=|-+  SaturateOnIntegerOverflow=on
  Sum1 : Sum  Inputs=|++  SaturateOnIntegerOverflow=on
  scaling : Gain  Gain=194/3.1678*.3684  SaturateOnIntegerOverflow=on  OutDataTypeStr=Inherit: Same as input  ParamDataTypeStr=Inherit: Same as input
  volts : Outport
  wires:
  Constant1/1 -> Sum1/2
  Sum1/1 -> volts/1
  scaling/1 -> Sum1/1
  raw/1 -> Sum/1
  Sum/1 -> scaling/1
  Constant/1 -> Sum/2

== system IOlib/Simulated Hardware/Simulated Driver/Automatic Manual Switch ==
  1 : Inport
  2 : Inport  Port=2
  3 : Inport  Port=3
  4 : Inport  Port=4
  Constant : Constant  Value=sw
  S-Function : S-Function  FunctionName=sfun_manswitch  Parameters=boolean(1)  EnableBusSupport=off
  Switch : Switch  Threshold=.5
  Switch1 : Switch  Threshold=.5
  Terminator : Terminator
  Out1 : Outport
  Out2 : Outport  Port=2
  wires:
  S-Function/1 -> Terminator/1
  Switch1/1 -> Out2/1
  4/1 -> Switch1/3
  3/1 -> Switch1/1
  Switch/1 -> Out1/1
  Constant/1 -> Switch1/2, Switch/2
  2/1 -> Switch/3
  1/1 -> Switch/1

== system IOlib/Simulated Hardware/Simulated Driver/Select: Speed ==
  In1 : Inport
  Gain : Gain  Gain=K  Multiplication=Matrix(K*u)  SaturateOnIntegerOverflow=on  OutDataTypeStr=Inherit: Same as input  ParamDataTypeStr=Inherit: Same as input
  Out1 : Outport
  wires:
  Gain/1 -> Out1/1
  In1/1 -> Gain/1

== system IOlib/Simulated Hardware/Steering System Model/Bicycle Model ==
  Steer Angles : Inport
  Vehicle Speed : Inport  Port=2
  State Adjust : Inport  Port=3
  Demux : Demux
  Demux1 : Demux  Outputs=2
  Demux2 : Demux  Outputs=2
  Demux3 : Demux  Outputs=2
  Mux2 : Mux  Inputs=7
  Rear Steer Angles : Ground
  S-Function : S-Function  FunctionName=bic_model  EnableBusSupport=off
  Yaw Rate : Outport
  Side-slip Angle : Outport  Port=2
  Left Tire Torque : Outport  Port=3
  Right Tire Torque : Outport  Port=4
  wires:
  S-Function/1 -> Demux/1
  Demux/3 -> Left Tire Torque/1
  Demux/4 -> Right Tire Torque/1
  Steer Angles/1 -> Demux3/1
  State Adjust/1 -> Demux1/1
  Mux2/1 -> S-Function/1
  Vehicle Speed/1 -> Mux2/1
  Demux3/1 -> Mux2/2
  Demux3/2 -> Mux2/3
  Demux/2 -> Yaw Rate/1
  Demux/1 -> Side-slip Angle/1
  Demux2/1 -> Mux2/4
  Demux2/2 -> Mux2/5
  Demux1/1 -> Mux2/6
  Demux1/2 -> Mux2/7
  Rear Steer Angles/1 -> Demux2/1

== system IOlib/Simulated Hardware/Steering System Model/Electrical Components and Motors ==
  Fault : Inport
  Steering Command : Inport  Port=2
  Torques : Inport  Port=3
  Amplifiers : Subsystem
      mask init:
      | amplifier_params
  Batteries : Subsystem  mask{v=50, vitf=tf([-50 -100],[1 110 1000])}
      mask prompts: v "Nominal voltage:"; vitf "Current-voltage transfer function:"
      mask init:
      | [vinum,viden]=tfdata(vitf);
      | vinum=vinum{1};
      | viden=viden{1};
  Demux2 : Demux  Outputs=2
  Motors : Subsystem
  Sum : Sum  SaturateOnIntegerOverflow=on
  Sensed Angles : Outport
  Motor Currents : Outport  Port=2
  Controller Currents : Outport  Port=3
  Battery Voltage : Outport  Port=4
  Motor Voltages : Outport  Port=5
  True Angles : Outport  Port=6
  wires:
  Motors/1(Angles) -> True Angles/1
  Torques/1 -> Motors/3(Load Torques)
  Steering Command/1 -> Amplifiers/3(Current Commands)
  Motors/2(Sensed Angles) -> Sensed Angles/1
  Fault/1 -> Motors/1(Fault)
  Motors/3(Currents) -> Amplifiers/2(Motor Currents), Motor Currents/1
  Amplifiers/2(Supply Currents) -> Controller Currents/1, Demux2/1
  Sum/1 -> Batteries/1(Current)
  Demux2/2 -> Sum/2
  Demux2/1 -> Sum/1
  Batteries/1(Voltage) -> Battery Voltage/1, Amplifiers/1(Supply Voltage)
  Amplifiers/1(Motor Voltages) -> Motors/2(Voltages), Motor Voltages/1

== system IOlib/Simulated Hardware/Steering System Model/Jacking Torques ==
  Motor Shaft Angles : Inport
  Demux1 : Demux  Outputs=2
  Gain : Gain  Gain=1/gr  SaturateOnIntegerOverflow=on  OutDataTypeStr=Inherit: Same as input  ParamDataTypeStr=Inherit: Same as input
  Left-hand look-up table : Lookup  InputValues=lma  Table=ljt  SaturateOnIntegerOverflow=on
  Mux6 : Mux  Inputs=2
  Right-hand look-up table : Lookup  InputValues=rma  Table=rjt  SaturateOnIntegerOverflow=on
  Jacking Torques : Outport
  wires:
  Right-hand look-up table/1 -> Mux6/2
  Demux1/2 -> Right-hand look-up table/1
  Left-hand look-up table/1 -> Mux6/1
  Mux6/1 -> Jacking Torques/1
  Demux1/1 -> Left-hand look-up table/1
  Gain/1 -> Demux1/1
  Motor Shaft Angles/1 -> Gain/1

== system IOlib/Simulated Hardware/Steering System Model/Mechanical Trail Change ==
  Motor Shaft Angles : Inport
  Nominal Aligning Torques : Inport  Port=2
  Demux1 : Demux  Outputs=2
  Gain : Gain  Gain=1/gr  SaturateOnIntegerOverflow=on  OutDataTypeStr=Inherit: Same as input  ParamDataTypeStr=Inherit: Same as input
  Gain1 : Gain  Gain=1/tm  SaturateOnIntegerOverflow=on  OutDataTypeStr=Inherit: Same as input  ParamDataTypeStr=Inherit: Same as input
  Left-hand look-up table : Lookup  InputValues=lma  Table=lmt  SaturateOnIntegerOverflow=on
  Mux6 : Mux  Inputs=2
  Product : Product  SaturateOnIntegerOverflow=on  OutDataTypeStr=Inherit: Same as first input
  Right-hand look-up table : Lookup  InputValues=rma  Table=rmt  SaturateOnIntegerOverflow=on
  Actual Aligning Torques : Outport
  wires:
  Mux6/1 -> Product/1
  Product/1 -> Actual Aligning Torques/1
  Gain1/1 -> Product/2
  Nominal Aligning Torques/1 -> Gain1/1
  Right-hand look-up table/1 -> Mux6/2
  Demux1/2 -> Right-hand look-up table/1
  Left-hand look-up table/1 -> Mux6/1
  Demux1/1 -> Left-hand look-up table/1
  Gain/1 -> Demux1/1
  Motor Shaft Angles/1 -> Gain/1

== system IOlib/Simulated Hardware/Steering System Model/Motor Shaft Angles to Steer Angles ==
  Motor Shaft Angles : Inport
  Demux1 : Demux  Outputs=2
  Gain : Gain  Gain=1/gr  SaturateOnIntegerOverflow=on  OutDataTypeStr=Inherit: Same as input  ParamDataTypeStr=Inherit: Same as input
  Left-hand look-up table : Lookup  InputValues=lma  Table=lsa  SaturateOnIntegerOverflow=on
  Mux6 : Mux  Inputs=2
  Right-hand look-up table : Lookup  InputValues=rma  Table=rsa  SaturateOnIntegerOverflow=on
  Steer Angles : Outport
  wires:
  Motor Shaft Angles/1 -> Gain/1
  Gain/1 -> Demux1/1
  Demux1/1 -> Left-hand look-up table/1
  Mux6/1 -> Steer Angles/1
  Left-hand look-up table/1 -> Mux6/1
  Demux1/2 -> Right-hand look-up table/1
  Right-hand look-up table/1 -> Mux6/2

== system IOlib/Fault Simulator/Input/Steering Motor Encoder Initialization/Left ==
  Encoder : Inport
  Potentiometer : Inport  Port=2
  Encoder Initializer : S-Function  FunctionName=encoderinit  Parameters=sampleTime,firstDelay,secondDelay  EnableBusSupport=off  mask{sampleTime=Ts, firstDelay=.1, secondDelay=.2}
      mask prompts: sampleTime "Sample time"; firstDelay "First calibration time"; secondDelay "Second calibration time"
      mask Display:
      | port_label('input',1,'Unwrapped');
      | port_label('input',2,'Raw');
      | port_label('input',3,'Pot');
      | port_label('output',1,'Calibrated');
  Unwrapper : S-Function  FunctionName=unwrapper  Parameters=Ts,2*pi  EnableBusSupport=off
      mask Display: disp('2*pi')
  Calibrated : Outport
  wires:
  Potentiometer/1 -> Encoder Initializer/3
  Unwrapper/1 -> Encoder Initializer/1
  Encoder/1 -> Unwrapper/1, Encoder Initializer/2
  Encoder Initializer/1 -> Calibrated/1

== system IOlib/Fault Simulator/Input/Steering Motor Encoder Initialization/Right ==
  Encoder : Inport
  Potentiometer : Inport  Port=2
  Encoder Initializer : S-Function  FunctionName=encoderinit  Parameters=sampleTime,firstDelay,secondDelay  EnableBusSupport=off  mask{sampleTime=Ts, firstDelay=.1, secondDelay=.2}
      mask prompts: sampleTime "Sample time"; firstDelay "First calibration time"; secondDelay "Second calibration time"
      mask Display:
      | port_label('input',1,'Unwrapped');
      | port_label('input',2,'Raw');
      | port_label('input',3,'Pot');
      | port_label('output',1,'Calibrated');
  Unwrapper : S-Function  FunctionName=unwrapper  Parameters=Ts,2*pi  EnableBusSupport=off
      mask Display: disp('2*pi')
  Calibrated : Outport
  wires:
  Encoder/1 -> Unwrapper/1, Encoder Initializer/2
  Unwrapper/1 -> Encoder Initializer/1
  Encoder Initializer/1 -> Calibrated/1
  Potentiometer/1 -> Encoder Initializer/3

== system IOlib/Simulated Hardware/Steering System Model/Electrical Components and Motors/Amplifiers ==
  Supply Voltage : Inport
  Motor Currents : Inport  Port=2
  Current Commands : Inport  Port=3
  Demux1 : Demux  Outputs=2
  Demux2 : Demux  Outputs=2
  Left Amplifier : Subsystem
  Mux1 : Mux  Inputs=2
  Mux5 : Mux  Inputs=2
  Right Amplifier : Subsystem
  Motor Voltages : Outport
  Supply Currents : Outport  Port=2
  wires:
  Right Amplifier/2(Supply Current) -> Mux1/2
  Left Amplifier/2(Supply Current) -> Mux1/1
  Right Amplifier/1(Motor Voltage) -> Mux5/2
  Left Amplifier/1(Motor Voltage) -> Mux5/1
  Demux1/2 -> Right Amplifier/3(Current Command)
  Demux1/1 -> Left Amplifier/3(Current Command)
  Demux2/2 -> Right Amplifier/2(Motor Current)
  Demux2/1 -> Left Amplifier/2(Motor Current)
  Supply Voltage/1 -> Right Amplifier/1(Supply Voltage), Left Amplifier/1(Supply Voltage)
  Mux1/1 -> Supply Currents/1
  Mux5/1 -> Motor Voltages/1
  Current Commands/1 -> Demux1/1
  Motor Currents/1 -> Demux2/1

== system IOlib/Simulated Hardware/Steering System Model/Electrical Components and Motors/Batteries ==
  Current : Inport
  Constant : Constant  Value=v
  Sum : Sum  Inputs=|++  SaturateOnIntegerOverflow=on
  Transfer Fcn : TransferFcn  Numerator=vinum  Denominator=viden
  Voltage : Outport
  wires:
  Sum/1 -> Voltage/1
  Current/1 -> Transfer Fcn/1
  Constant/1 -> Sum/2
  Transfer Fcn/1 -> Sum/1

== system IOlib/Simulated Hardware/Steering System Model/Electrical Components and Motors/Motors ==
  Fault : Inport
  Voltages : Inport  Port=2
  Load Torques : Inport  Port=3
  Demux1 : Demux  Outputs=2
  Demux2 : Demux  Outputs=2
  Demux3 : Demux
  Direct Look-Up Table (n-D) : LookupNDDirect  InputsSelectThisObjectFromTable=Column  Table=[0 1 0 0 0 0; 0 0 0 14 0 0; 0 0 1 0 0 0; 0 0 0 0 14 0]
  Left Motor : Subsystem  mask{vparams=p1_params.m}
      mask prompts: vparams "Vehicle parameters file"
      mask init:
      | % Load vehicle parameters file
      | evalc(strrep(vparams,'.m',''));
  Mux1 : Mux  Inputs=2
  Mux2 : Mux  Inputs=2
  Mux5 : Mux  Inputs=2
  Right Motor : Subsystem  mask{vparams=p1_params.m}
      mask prompts: vparams "Vehicle parameters file"
      mask init:
      | % Load vehicle parameters file
      | evalc(strrep(vparams,'.m',''));
  Sum1 : Sum  Inputs=++|  SaturateOnIntegerOverflow=on
  Angles : Outport
  Sensed Angles : Outport  Port=2
  Currents : Outport  Port=3
  wires:
  Sum1/1 -> Sensed Angles/1
  Mux2/1 -> Sum1/2
  Demux3/4 -> Mux2/2
  Demux3/2 -> Mux2/1
  Demux3/3 -> Right Motor/1(Fault)
  Demux3/1 -> Left Motor/1(Fault)
  Fault/1 -> Direct Look-Up Table (n-D)/1
  Direct Look-Up Table (n-D)/1 -> Demux3/1
  Mux1/1 -> Currents/1
  Mux5/1 -> Sum1/1, Angles/1
  Right Motor/2(Current) -> Mux1/2
  Left Motor/2(Current) -> Mux1/1
  Right Motor/1(Angle) -> Mux5/2
  Left Motor/1(Angle) -> Mux5/1
  Demux1/2 -> Right Motor/3(Load Torque)
  Demux1/1 -> Left Motor/3(Load Torque)
  Demux2/2 -> Right Motor/2(Voltage)
  Demux2/1 -> Left Motor/2(Voltage)
  Load Torques/1 -> Demux1/1
  Voltages/1 -> Demux2/1

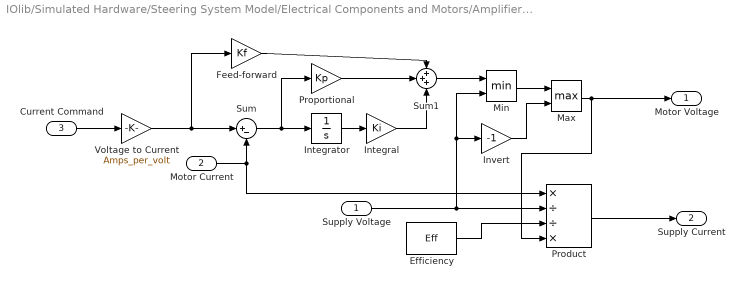
== system IOlib/Simulated Hardware/Steering System Model/Electrical Components and Motors/Amplifiers/Left Amplifier ==
  Supply Voltage : Inport
  Motor Current : Inport  Port=2
  Current Command : Inport  Port=3
  Efficiency : Constant  Value=Eff
  Feed-forward : Gain  Gain=Kf  SaturateOnIntegerOverflow=on  OutDataTypeStr=Inherit: Same as input  ParamDataTypeStr=Inherit: Same as input
  Integral : Gain  Gain=Ki  SaturateOnIntegerOverflow=on  OutDataTypeStr=Inherit: Same as input  ParamDataTypeStr=Inherit: Same as input
  Integrator : Integrator
  Invert : Gain  Gain=-1  SaturateOnIntegerOverflow=on  OutDataTypeStr=Inherit: Same as input  ParamDataTypeStr=Inherit: Same as input
  Max : MinMax  Function=max  Inputs=2  ZeroCross=off  SaturateOnIntegerOverflow=on  InputSameDT=on
  Min : MinMax  Inputs=2  ZeroCross=off  SaturateOnIntegerOverflow=on  InputSameDT=on
  Product : Product  Inputs=*//*  SaturateOnIntegerOverflow=on  OutDataTypeStr=Inherit: Same as first input
  Proportional : Gain  Gain=Kp  SaturateOnIntegerOverflow=on  OutDataTypeStr=Inherit: Same as input  ParamDataTypeStr=Inherit: Same as input
  Sum : Sum  Inputs=|+-  SaturateOnIntegerOverflow=on
  Sum1 : Sum  Inputs=+++  SaturateOnIntegerOverflow=on
  Voltage to Current : Gain  Gain=Amps_per_volt  SaturateOnIntegerOverflow=on  OutDataTypeStr=Inherit: Same as input  ParamDataTypeStr=Inherit: Same as input
  Motor Voltage : Outport
  Supply Current : Outport  Port=2
  wires:
  Current Command/1 -> Voltage to Current/1
  Voltage to Current/1 -> Feed-forward/1, Sum/1
  Motor Current/1 -> Product/1, Sum/2
  Efficiency/1 -> Product/3
  Sum1/1 -> Min/1
  Product/1 -> Supply Current/1
  Sum/1 -> Integrator/1, Proportional/1
  Integrator/1 -> Integral/1
  Integral/1 -> Sum1/3
  Proportional/1 -> Sum1/2
  Feed-forward/1 -> Sum1/1
  Supply Voltage/1 -> Product/2, Min/2, Invert/1
  Max/1 -> Motor Voltage/1, Product/4
  Min/1 -> Max/1
  Invert/1 -> Max/2

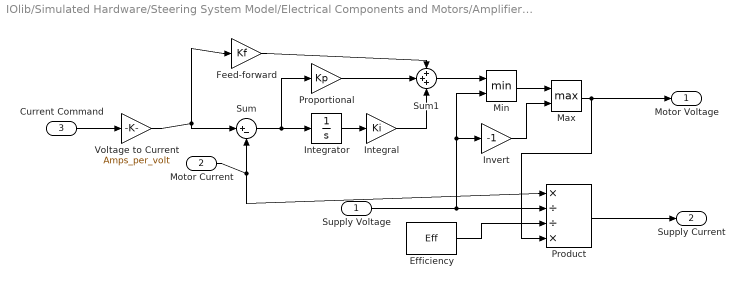
== system IOlib/Simulated Hardware/Steering System Model/Electrical Components and Motors/Amplifiers/Right Amplifier ==
  Supply Voltage : Inport
  Motor Current : Inport  Port=2
  Current Command : Inport  Port=3
  Efficiency : Constant  Value=Eff
  Feed-forward : Gain  Gain=Kf  SaturateOnIntegerOverflow=on  OutDataTypeStr=Inherit: Same as input  ParamDataTypeStr=Inherit: Same as input
  Integral : Gain  Gain=Ki  SaturateOnIntegerOverflow=on  OutDataTypeStr=Inherit: Same as input  ParamDataTypeStr=Inherit: Same as input
  Integrator : Integrator
  Invert : Gain  Gain=-1  SaturateOnIntegerOverflow=on  OutDataTypeStr=Inherit: Same as input  ParamDataTypeStr=Inherit: Same as input
  Max : MinMax  Function=max  Inputs=2  ZeroCross=off  SaturateOnIntegerOverflow=on  InputSameDT=on
  Min : MinMax  Inputs=2  ZeroCross=off  SaturateOnIntegerOverflow=on  InputSameDT=on
  Product : Product  Inputs=*//*  SaturateOnIntegerOverflow=on  OutDataTypeStr=Inherit: Same as first input
  Proportional : Gain  Gain=Kp  SaturateOnIntegerOverflow=on  OutDataTypeStr=Inherit: Same as input  ParamDataTypeStr=Inherit: Same as input
  Sum : Sum  Inputs=|+-  SaturateOnIntegerOverflow=on
  Sum1 : Sum  Inputs=+++  SaturateOnIntegerOverflow=on
  Voltage to Current : Gain  Gain=Amps_per_volt  SaturateOnIntegerOverflow=on  OutDataTypeStr=Inherit: Same as input  ParamDataTypeStr=Inherit: Same as input
  Motor Voltage : Outport
  Supply Current : Outport  Port=2
  wires:
  Invert/1 -> Max/2
  Min/1 -> Max/1
  Max/1 -> Product/4, Motor Voltage/1
  Supply Voltage/1 -> Invert/1, Min/2, Product/2
  Feed-forward/1 -> Sum1/1
  Proportional/1 -> Sum1/2
  Integral/1 -> Sum1/3
  Integrator/1 -> Integral/1
  Sum/1 -> Proportional/1, Integrator/1
  Product/1 -> Supply Current/1
  Sum1/1 -> Min/1
  Efficiency/1 -> Product/3
  Motor Current/1 -> Sum/2, Product/1
  Voltage to Current/1 -> Sum/1, Feed-forward/1
  Current Command/1 -> Voltage to Current/1
